simulink model "IFSSIM_Aero"  (R2025b)
settings: Solver=FixedStepDiscrete  StartTime=0  StopTime=inf  FixedStep=1/960  RelTol=1e-3
settings Model: Creator=raulmoran  LastModifiedBy=raulmoran

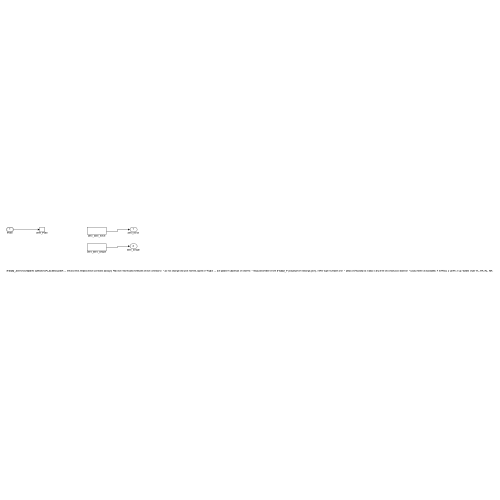
[thumbnail: Simulink's stored preview of the top-level diagram]
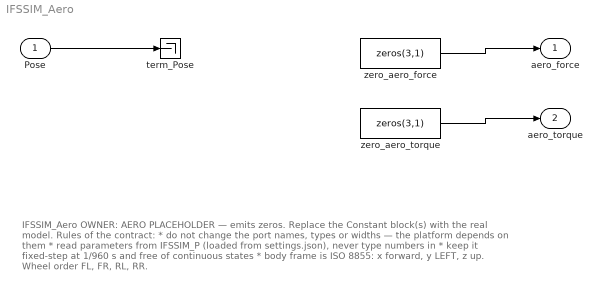
== system IFSSIM_Aero ==
  note: IFSSIM_Aero\n\nOWNER: AERO\n\nPLACEHOLDER — emits zeros. Replace the Constant block(s) with the real model.\n\nRules of the contract:\n * do not change the port names, types or widths — the platform depends on them\n * read parameters from IFSSIM_P (loaded from settings.json), never type numbers in\n * keep it fixed-step at 1/960 s and free of continuous states\n * body frame is ISO 8855: x forward, y LEFT, z up. Wheel order FL, FR, RL, RR.
  Pose : Inport  OutDataTypeStr=Bus: IFSSIM_PoseBus  BusOutputAsStruct=on
  term_Pose : Terminator
  zero_aero_force : Constant  Value=zeros(3,1)
  zero_aero_torque : Constant  Value=zeros(3,1)
  aero_force : Outport  PortDimensions=3
  aero_torque : Outport  Port=2  PortDimensions=3
  wires:
  Pose/1 -> term_Pose/1
  zero_aero_force/1 -> aero_force/1
  zero_aero_torque/1 -> aero_torque/1
